simulink model "servopositioner"  (R2015b)
settings: Solver=ode45  StartTime=0.0  StopTime=100  RelTol=1e-3
values from neighbouring files (symbols this model uses):
  Aa = pi*(Dp^2)/4    (= 0.00020106192983)    [param_JOB.m]
  Ab = pi*(Dp^2-Dr^2)/4    (= 0.00012252211349)    [param_JOB.m]
  acc = 0    [param_JOB.m]
  beta = 1.4e9    (= 1400000000)    [param_JOB.m]
  fv = 700    [param_JOB.m]
  In = 10e-3    (= 0.01)    [param_JOB.m]
  Kva = Kv*sqrt(2)    [param_JOB.m]
  Kvb = Kv*sqrt(2)    [param_JOB.m]
  KvlkA = Kvlk    [param_JOB.m]
  KvlkB = Kvlk    [param_JOB.m]
  L = 0.5    [beta_hose_calc.m]    (also in param_JOB.m = 0.08)
  leak = 0    [param_JOB.m]
  lw_dz = 0    [param_JOB.m]
  Mp = ((pi*Dr^2/4)*L + Aa*0.15)*7860    (= 0.286437851784)    [param_JOB.m]
  n = 1.4    [beta_hose_calc.m]    (also in beta_w_air_entrance.m; param_JOB.m)
  P0 = 100e5    (= 10000000)    [beta_hose_calc.m]    (also in param_JOB.m)
  pAo = ps/2    (= 8000000)    [param_JOB.m]
  pBo = ps/2    (= 8000000)    [param_JOB.m]
  ps = 1e5:1e5:120e5    [beta_w_air_entrance.m]    (also in param_JOB.m = 16000000)
  pt = 10e5    (= 1000000)    [param_JOB.m]
  up_dz = 0    [param_JOB.m]
  V0 = A*L    (= 6.13592315154e-05)    [beta_hose_calc.m]    (also in param_JOB.m = 4e-05)
  V0A = v1a + v2a    (= 2.90341084306e-06)    [param_JOB.m]
  V0B = v1b + v2b + v3b    (= 1.67615552692e-06)    [param_JOB.m]
  wn = 2*100*pi    (= 628.318530718)    [param_JOB.m]
libraries: simulink x2
settings Model: Creator=Toshiba  LastModifiedBy=Toshiba
settings SolverCC: ZeroCrossAlgorithm=Adaptive
settings DataIOCC: SaveFormat=Array
settings DebuggingCC: UnderspecifiedInitializationDetection=Classic  MergeDetectMultiDrivingBlocksExec=none  SolverPrmCheckMsg=warning  StateNameClashWarn=warning
settings HardwareCC: ProdBitPerPointer=32  ProdLargestAtomicFloat=None  ProdIntDivRoundTo=Undefined  ProdEndianess=Unspecified  ProdWordSize=32  ProdHWDeviceType=32-bit Generic
settings GRTTargetCC: GeneratePreprocessorConditionals=Disable all
settings ConfigComp: CovModelRefEnable=Off

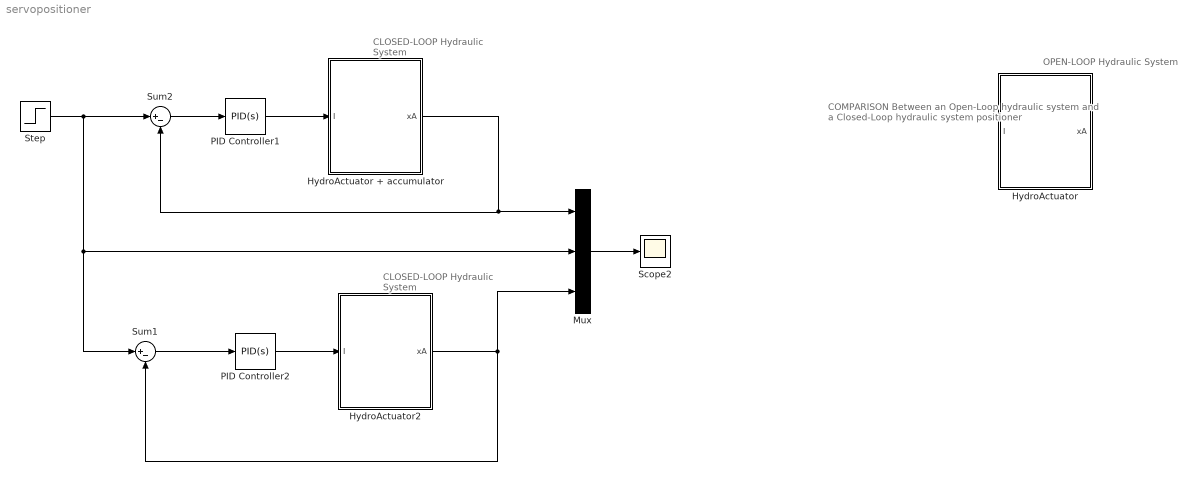
== system servopositioner ==
  note: OPEN-LOOP
      | Hydraulic System
  note: COMPARISON Between
      | an Open-Loop hydraulic system
      | and a Closed-Loop hydraulic
      | system positioner
  note: CLOSED-LOOP
      | Hydraulic System
  note: CLOSED-LOOP
      | Hydraulic System
  HydroActuator : Subsystem
  HydroActuator + accumulator : Subsystem
  HydroActuator2 : Subsystem
  Mux : Mux  Inputs=3
  PID Controller1 : simulink/Continuous/PID Controller  Controller=PID  TimeDomain=Continuous-time  SampleTime=-1  IntegratorMethod=Forward Euler  FilterMethod=Forward Euler  Form=Parallel  UseFilter=on  ControllerParametersSource=internal  P=700  I=50  D=0  N=100  InitialConditionSource=internal  InitialConditionForIntegrator=0  InitialConditionForFilter=0  ExternalReset=none  LimitOutput=off  UpperSaturationLimit=inf  LowerSaturationLimit=-inf  LinearizeAsGain=on  AntiWindupMode=none  Kb=1  TrackingMode=off  Kt=1  PParamMin=[]  PParamMax=[]  IParamMin=[]  IParamMax=[]  DParamMin=[]  DParamMax=[]  NParamMin=[]  NParamMax=[]  KbParamMin=[]  KbParamMax=[]  KtParamMin=[]  KtParamMax=[]  POutMin=[]  POutMax=[]  IOutMin=[]  IOutMax=[]  DOutMin=[]  DOutMax=[]  NOutMin=[]  NOutMax=[]  KbOutMin=[]  KbOutMax=[]  KtOutMin=[]  KtOutMax=[]  IntegratorOutMin=[]  IntegratorOutMax=[]  FilterOutMin=[]  FilterOutMax=[]  SumOutMin=[]  SumOutMax=[]  SumI1OutMin=[]  SumI1OutMax=[]  SumI2OutMin=[]  SumI2OutMax=[]  SumI3OutMin=[]  SumI3OutMax=[]  SumDOutMin=[]  SumDOutMax=[]  SaturationOutMin=[]  SaturationOutMax=[]  IntegratorContinuousStateAttributes=''  IntegratorStateMustResolveToSignalObject=off  IntegratorRTWStateStorageClass=Auto  FilterContinuousStateAttributes=''  FilterStateMustResolveToSignalObject=off  FilterRTWStateStorageClass=Auto  DifferentiatorICPrevScaledInput=0  DifferentiatorOutMin=[]  DifferentiatorOutMax=[]
  PID Controller2 : simulink/Continuous/PID Controller  Controller=PID  TimeDomain=Continuous-time  SampleTime=-1  IntegratorMethod=Forward Euler  FilterMethod=Forward Euler  Form=Parallel  UseFilter=on  ControllerParametersSource=internal  P=700  I=50  D=0  N=100  InitialConditionSource=internal  InitialConditionForIntegrator=0  InitialConditionForFilter=0  ExternalReset=none  LimitOutput=off  UpperSaturationLimit=inf  LowerSaturationLimit=-inf  LinearizeAsGain=on  AntiWindupMode=none  Kb=1  TrackingMode=off  Kt=1  PParamMin=[]  PParamMax=[]  IParamMin=[]  IParamMax=[]  DParamMin=[]  DParamMax=[]  NParamMin=[]  NParamMax=[]  KbParamMin=[]  KbParamMax=[]  KtParamMin=[]  KtParamMax=[]  POutMin=[]  POutMax=[]  IOutMin=[]  IOutMax=[]  DOutMin=[]  DOutMax=[]  NOutMin=[]  NOutMax=[]  KbOutMin=[]  KbOutMax=[]  KtOutMin=[]  KtOutMax=[]  IntegratorOutMin=[]  IntegratorOutMax=[]  FilterOutMin=[]  FilterOutMax=[]  SumOutMin=[]  SumOutMax=[]  SumI1OutMin=[]  SumI1OutMax=[]  SumI2OutMin=[]  SumI2OutMax=[]  SumI3OutMin=[]  SumI3OutMax=[]  SumDOutMin=[]  SumDOutMax=[]  SaturationOutMin=[]  SaturationOutMax=[]  IntegratorContinuousStateAttributes=''  IntegratorStateMustResolveToSignalObject=off  IntegratorRTWStateStorageClass=Auto  FilterContinuousStateAttributes=''  FilterStateMustResolveToSignalObject=off  FilterRTWStateStorageClass=Auto  DifferentiatorICPrevScaledInput=0  DifferentiatorOutMin=[]  DifferentiatorOutMax=[]
  Scope2 : Scope
  Step : Step  Time=3  After=0.04  SampleTime=0
  Sum1 : Sum  Inputs=|+-
  Sum2 : Sum  Inputs=|+-
  wires:
  Step/1 -> Sum2/1, Mux/2, Sum1/1
  PID Controller1/1 -> HydroActuator + accumulator/1(I)
  Mux/1 -> Scope2/1
  HydroActuator2/1(xA) -> Mux/3, Sum1/2
  Sum1/1 -> PID Controller2/1
  PID Controller2/1 -> HydroActuator2/1(I)
  Sum2/1 -> PID Controller1/1
  HydroActuator + accumulator/1(xA) -> Sum2/2, Mux/1

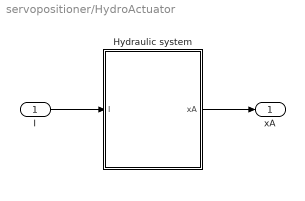
== system servopositioner/HydroActuator ==
  I : Inport
  Hydraulic system : Subsystem
  xA : Outport
  wires:
  I/1 -> Hydraulic system/1(I)
  Hydraulic system/1(xA) -> xA/1

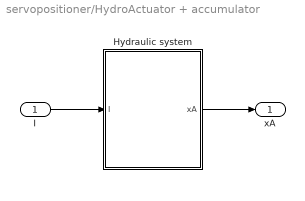
== system servopositioner/HydroActuator + accumulator ==
  I : Inport
  Hydraulic system : Subsystem
  xA : Outport
  wires:
  Hydraulic system/1(xA) -> xA/1
  I/1 -> Hydraulic system/1(I)

== system servopositioner/HydroActuator2 ==
  I : Inport
  Hydraulic system : Subsystem
  xA : Outport
  wires:
  I/1 -> Hydraulic system/1(I)
  Hydraulic system/1(xA) -> xA/1

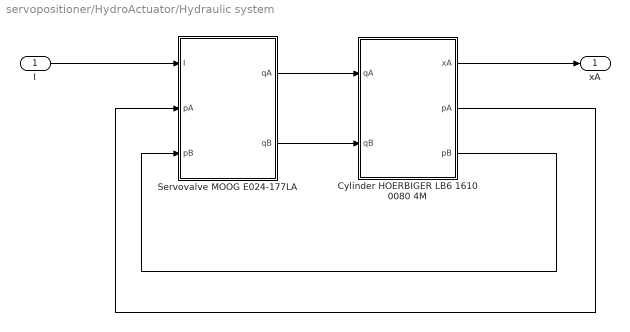
== system servopositioner/HydroActuator/Hydraulic system ==
  I : Inport
  Cylinder HOERBIGER LB6 1610 0080 4M : Subsystem
  Servovalve MOOG E024-177LA : Subsystem
  xA : Outport
  wires:
  Servovalve MOOG E024-177LA/2(qB) -> Cylinder HOERBIGER LB6 1610 0080 4M/2(qB)
  Servovalve MOOG E024-177LA/1(qA) -> Cylinder HOERBIGER LB6 1610 0080 4M/1(qA)
  Cylinder HOERBIGER LB6 1610 0080 4M/2(pA) -> Servovalve MOOG E024-177LA/2(pA)
  Cylinder HOERBIGER LB6 1610 0080 4M/3(pB) -> Servovalve MOOG E024-177LA/3(pB)
  I/1 -> Servovalve MOOG E024-177LA/1(I)
  Cylinder HOERBIGER LB6 1610 0080 4M/1(xA) -> xA/1

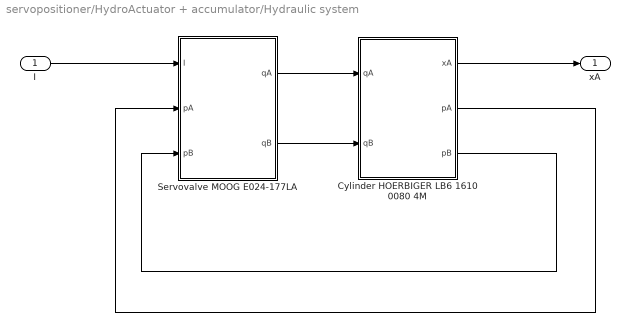
== system servopositioner/HydroActuator + accumulator/Hydraulic system ==
  I : Inport
  Cylinder HOERBIGER LB6 1610 0080 4M : Subsystem
  Servovalve MOOG E024-177LA : Subsystem
  xA : Outport
  wires:
  Cylinder HOERBIGER LB6 1610 0080 4M/1(xA) -> xA/1
  I/1 -> Servovalve MOOG E024-177LA/1(I)
  Cylinder HOERBIGER LB6 1610 0080 4M/3(pB) -> Servovalve MOOG E024-177LA/3(pB)
  Cylinder HOERBIGER LB6 1610 0080 4M/2(pA) -> Servovalve MOOG E024-177LA/2(pA)
  Servovalve MOOG E024-177LA/1(qA) -> Cylinder HOERBIGER LB6 1610 0080 4M/1(qA)
  Servovalve MOOG E024-177LA/2(qB) -> Cylinder HOERBIGER LB6 1610 0080 4M/2(qB)

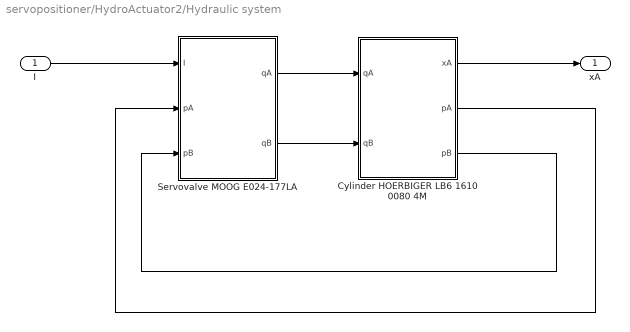
== system servopositioner/HydroActuator2/Hydraulic system ==
  I : Inport
  Cylinder HOERBIGER LB6 1610 0080 4M : Subsystem
  Servovalve MOOG E024-177LA : Subsystem
  xA : Outport
  wires:
  Servovalve MOOG E024-177LA/2(qB) -> Cylinder HOERBIGER LB6 1610 0080 4M/2(qB)
  Servovalve MOOG E024-177LA/1(qA) -> Cylinder HOERBIGER LB6 1610 0080 4M/1(qA)
  Cylinder HOERBIGER LB6 1610 0080 4M/2(pA) -> Servovalve MOOG E024-177LA/2(pA)
  Cylinder HOERBIGER LB6 1610 0080 4M/3(pB) -> Servovalve MOOG E024-177LA/3(pB)
  I/1 -> Servovalve MOOG E024-177LA/1(I)
  Cylinder HOERBIGER LB6 1610 0080 4M/1(xA) -> xA/1

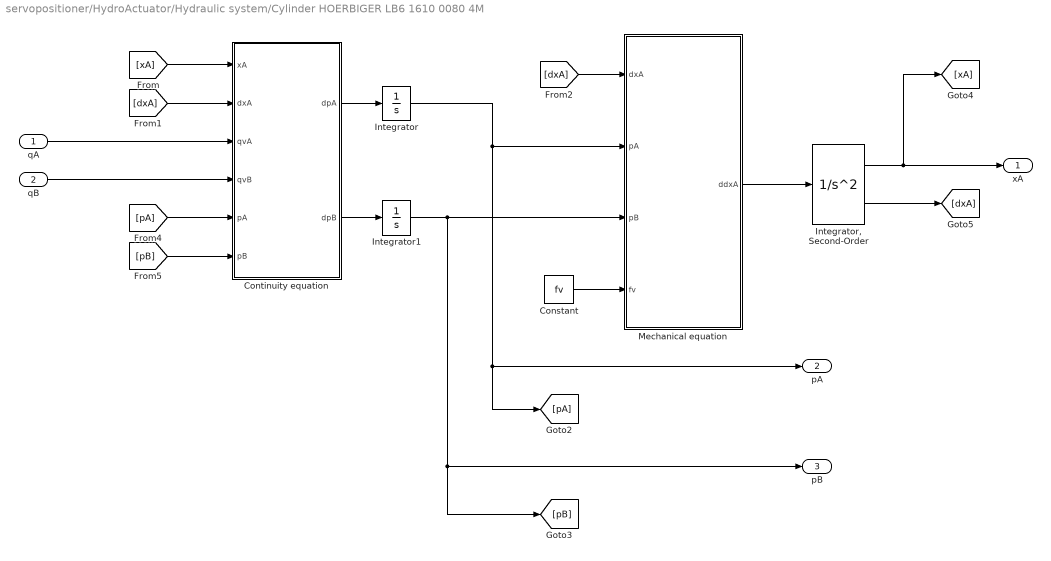
== system servopositioner/HydroActuator/Hydraulic system/Cylinder HOERBIGER LB6 1610 0080 4M ==
  qA : Inport
  qB : Inport  Port=2
  Constant : Constant  Value=fv
  Continuity equation : MATLAB Function  TreatAsAtomicUnit=on
  Integrator : Integrator  InitialCondition=pAo
  "Integrator, Second-Order" : SecondOrderIntegrator  ICX=xo  LimitX=on  UpperLimitX=L  LowerLimitX=0
  Integrator1 : Integrator  InitialCondition=pBo
  Mechanical equation : MATLAB Function  TreatAsAtomicUnit=on
  xA : Outport
  pA : Outport  Port=2
  pB : Outport  Port=3
  wires:
  Continuity equation/1(dpA) -> Integrator/1
  Continuity equation/2(dpB) -> Integrator1/1
  qA/1 -> Continuity equation/3(qvA)
  qB/1 -> Continuity equation/4(qvB)
  [dxA] -> Continuity equation/2(dxA)
  [xA] -> Continuity equation/1(xA)
  Constant/1 -> Mechanical equation/4(fv)
  [dxA] -> Mechanical equation/1(dxA)
  Integrator/1 -> [pA], pA/1, Mechanical equation/2(pA)
  Integrator1/1 -> [pB], pB/1, Mechanical equation/3(pB)
  [pA] -> Continuity equation/5(pA)
  [pB] -> Continuity equation/6(pB)
  Mechanical equation/1(ddxA) -> "Integrator, Second-Order"/1
  "Integrator, Second-Order"/1 -> xA/1, [xA]
  "Integrator, Second-Order"/2 -> [dxA]

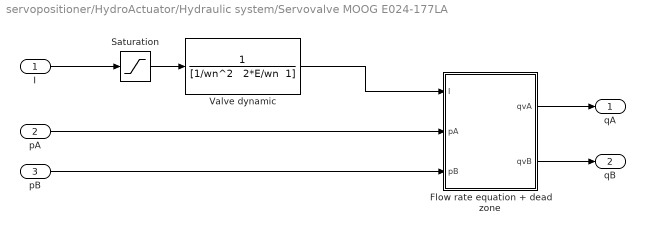
== system servopositioner/HydroActuator/Hydraulic system/Servovalve MOOG E024-177LA ==
  I : Inport
  pA : Inport  Port=2
  pB : Inport  Port=3
  Flow rate equation + dead zone : MATLAB Function  TreatAsAtomicUnit=on
  Saturation : Saturate  UpperLimit=In  LowerLimit=-In  LinearizeAsGain=off
  Valve dynamic : TransferFcn  Numerator=1  Denominator="[1/wn^2   2*E/wn  1]"
  qA : Outport
  qB : Outport  Port=2
  wires:
  Saturation/1 -> Valve dynamic/1
  I/1 -> Saturation/1
  Valve dynamic/1 -> Flow rate equation + dead zone/1(I)
  pA/1 -> Flow rate equation + dead zone/2(pA)
  pB/1 -> Flow rate equation + dead zone/3(pB)
  Flow rate equation + dead zone/2(qvB) -> qB/1
  Flow rate equation + dead zone/1(qvA) -> qA/1

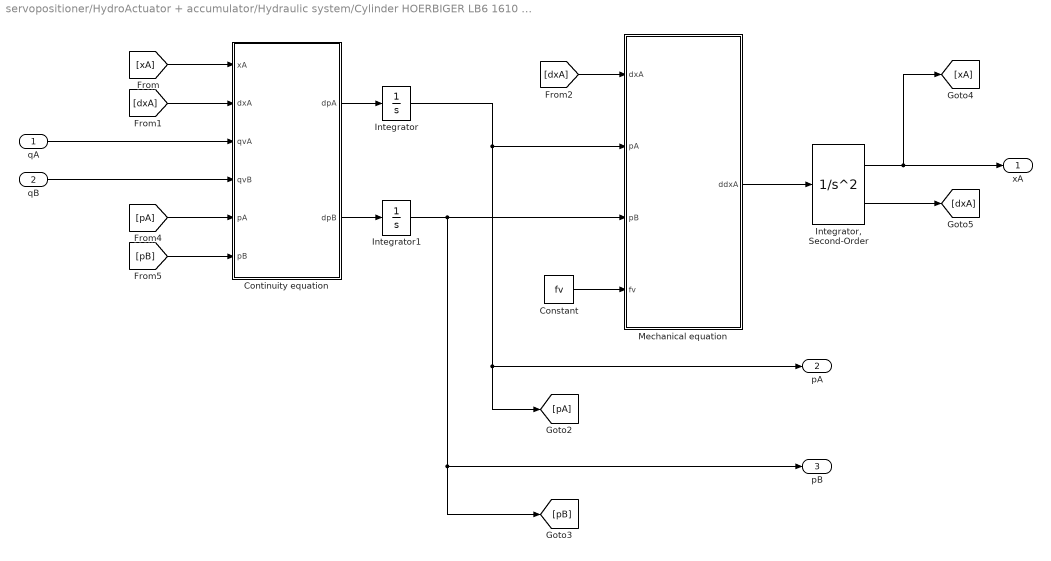
== system servopositioner/HydroActuator + accumulator/Hydraulic system/Cylinder HOERBIGER LB6 1610 0080 4M ==
  qA : Inport
  qB : Inport  Port=2
  Constant : Constant  Value=fv
  Continuity equation : MATLAB Function  TreatAsAtomicUnit=on
  Integrator : Integrator  InitialCondition=pAo
  "Integrator, Second-Order" : SecondOrderIntegrator  ICX=xo  LimitX=on  UpperLimitX=L  LowerLimitX=0
  Integrator1 : Integrator  InitialCondition=pBo
  Mechanical equation : MATLAB Function  TreatAsAtomicUnit=on
  xA : Outport
  pA : Outport  Port=2
  pB : Outport  Port=3
  wires:
  "Integrator, Second-Order"/2 -> [dxA]
  "Integrator, Second-Order"/1 -> [xA], xA/1
  Mechanical equation/1(ddxA) -> "Integrator, Second-Order"/1
  [pB] -> Continuity equation/6(pB)
  [pA] -> Continuity equation/5(pA)
  Integrator1/1 -> Mechanical equation/3(pB), pB/1, [pB]
  Integrator/1 -> Mechanical equation/2(pA), pA/1, [pA]
  [dxA] -> Mechanical equation/1(dxA)
  Constant/1 -> Mechanical equation/4(fv)
  [xA] -> Continuity equation/1(xA)
  [dxA] -> Continuity equation/2(dxA)
  qB/1 -> Continuity equation/4(qvB)
  qA/1 -> Continuity equation/3(qvA)
  Continuity equation/2(dpB) -> Integrator1/1
  Continuity equation/1(dpA) -> Integrator/1

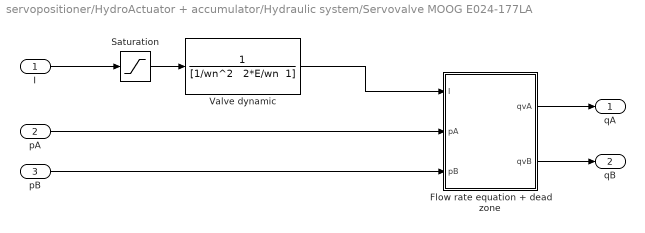
== system servopositioner/HydroActuator + accumulator/Hydraulic system/Servovalve MOOG E024-177LA ==
  I : Inport
  pA : Inport  Port=2
  pB : Inport  Port=3
  Flow rate equation + dead zone : MATLAB Function  TreatAsAtomicUnit=on
  Saturation : Saturate  UpperLimit=In  LowerLimit=-In  LinearizeAsGain=off
  Valve dynamic : TransferFcn  Numerator=1  Denominator="[1/wn^2   2*E/wn  1]"
  qA : Outport
  qB : Outport  Port=2
  wires:
  Flow rate equation + dead zone/1(qvA) -> qA/1
  Flow rate equation + dead zone/2(qvB) -> qB/1
  pB/1 -> Flow rate equation + dead zone/3(pB)
  pA/1 -> Flow rate equation + dead zone/2(pA)
  Valve dynamic/1 -> Flow rate equation + dead zone/1(I)
  I/1 -> Saturation/1
  Saturation/1 -> Valve dynamic/1

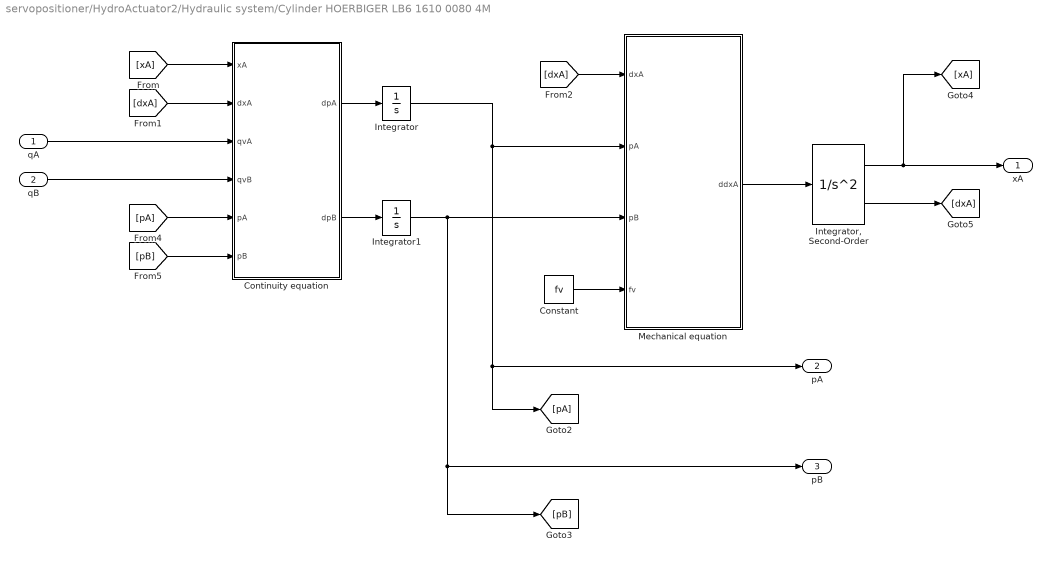
== system servopositioner/HydroActuator2/Hydraulic system/Cylinder HOERBIGER LB6 1610 0080 4M ==
  qA : Inport
  qB : Inport  Port=2
  Constant : Constant  Value=fv
  Continuity equation : MATLAB Function  TreatAsAtomicUnit=on
  Integrator : Integrator  InitialCondition=pAo
  "Integrator, Second-Order" : SecondOrderIntegrator  ICX=xo  LimitX=on  UpperLimitX=L  LowerLimitX=0
  Integrator1 : Integrator  InitialCondition=pBo
  Mechanical equation : MATLAB Function  TreatAsAtomicUnit=on
  xA : Outport
  pA : Outport  Port=2
  pB : Outport  Port=3
  wires:
  Continuity equation/1(dpA) -> Integrator/1
  Continuity equation/2(dpB) -> Integrator1/1
  qA/1 -> Continuity equation/3(qvA)
  qB/1 -> Continuity equation/4(qvB)
  [dxA] -> Continuity equation/2(dxA)
  [xA] -> Continuity equation/1(xA)
  Constant/1 -> Mechanical equation/4(fv)
  [dxA] -> Mechanical equation/1(dxA)
  Integrator/1 -> [pA], pA/1, Mechanical equation/2(pA)
  Integrator1/1 -> [pB], pB/1, Mechanical equation/3(pB)
  [pA] -> Continuity equation/5(pA)
  [pB] -> Continuity equation/6(pB)
  Mechanical equation/1(ddxA) -> "Integrator, Second-Order"/1
  "Integrator, Second-Order"/1 -> xA/1, [xA]
  "Integrator, Second-Order"/2 -> [dxA]

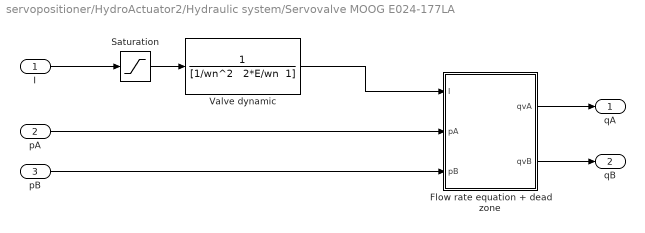
== system servopositioner/HydroActuator2/Hydraulic system/Servovalve MOOG E024-177LA ==
  I : Inport
  pA : Inport  Port=2
  pB : Inport  Port=3
  Flow rate equation + dead zone : MATLAB Function  TreatAsAtomicUnit=on
  Saturation : Saturate  UpperLimit=In  LowerLimit=-In  LinearizeAsGain=off
  Valve dynamic : TransferFcn  Numerator=1  Denominator="[1/wn^2   2*E/wn  1]"
  qA : Outport
  qB : Outport  Port=2
  wires:
  Saturation/1 -> Valve dynamic/1
  I/1 -> Saturation/1
  Valve dynamic/1 -> Flow rate equation + dead zone/1(I)
  pA/1 -> Flow rate equation + dead zone/2(pA)
  pB/1 -> Flow rate equation + dead zone/3(pB)
  Flow rate equation + dead zone/2(qvB) -> qB/1
  Flow rate equation + dead zone/1(qvA) -> qA/1

== matlab function servopositioner/HydroActuator + accumulator/Hydraulic system/Cylinder HOERBIGER LB6 1610 0080 4M/Continuity equation ==
  data: xA input; dpA output; dpB output; dxA input; qvA input; qvB input; pA input; pB input; leak parameter; V0A parameter; V0B parameter; Aa parameter; Ab parameter; L parameter; beta parameter; n parameter; V0 parameter; P0 parameter
function [dpA,dpB] = fcn(xA, dxA, qvA, qvB, pA, pB, leak, V0A, V0B, Aa, Ab, L, beta, n, V0, P0)

pC = pA - pB;   % Pressao de carga [Pa]

qvlk = leak * pC;
  
CA_A  = (V0A + Aa*xA) / beta;                      % Capacitancia hidráulica do atuador [m^3/Pa]
CAC_A = (V0*P0^(1/n))/(n* (pA+1e5)^((n+1)/n));     % Capacitancia hidráulica do acumulador [m^3/Pa]
CA_B  = (V0B + Ab*(L-xA)) / beta;                  % Capacitancia hidráulica do atuador [m^3/Pa]
CAC_B = (V0*P0^(1/n))/(n* (pB+1e5)^((n+1)/n));     % Capacitancia hidráulica do acumulador [m^3/Pa]

CT_A  = CA_A + CAC_A;                              % Capacitancia total em A
CT_B  = CA_B + CAC_B;                              % Capacitancia total em B 

%       /        \
%       |   1    | /                    \
% dpA = | ------ | | qvA - Aa*dx - qvex | 
%       |  CT_A  | \                    /
%       \        /
      
dpA = CT_A^-1 * (qvA - Aa*dxA - qvlk);

%       /        \
%       |   1    | /                    \
% dpB = | ------ | | Ab*dx + qvex - qvB | 
%       |  CT_B  | \                    /
%       \        /
      
dpB = CT_B^-1 * (Ab*dxA + qvlk - qvB);

== matlab function servopositioner/HydroActuator + accumulator/Hydraulic system/Cylinder HOERBIGER LB6 1610 0080 4M/Mechanical equation ==
  data: ddxA output; dxA input; pA input; pB input; fv input; Aa parameter; Ab parameter; Mp parameter
function ddxA = fcn(dxA, pA, pB, fv, Aa, Ab, Mp)
%#codegen

FH  = pA*Aa - pB*Ab;     % N - Hydraulic force
Ffr = fv*dxA;            % N - Friction force (Viscous)
ddxA  = (FH - Ffr)/Mp;     % m/s2 - Acceleration

== matlab function servopositioner/HydroActuator/Hydraulic system/Cylinder HOERBIGER LB6 1610 0080 4M/Continuity equation ==
  data: xA input; dpA output; dpB output; dxA input; qvA input; qvB input; pA input; pB input; leak parameter; V0A parameter; V0B parameter; Aa parameter; Ab parameter; L parameter; beta parameter; n parameter; V0 parameter; P0 parameter; acc parameter
function [dpA,dpB] = fcn(xA, dxA, qvA, qvB, pA, pB, leak, V0A, V0B, Aa, Ab, L, beta, n, V0, P0, acc)

pC = pA - pB;   % Pressao de carga [Pa]

qvlk = leak * pC;
dpa = 0;
dpb = 0;

if acc == 0,
%       /              \
%       |     beta     | /                    \
% dpA = | ------------ | | qvA - Aa*dx - qvex | 
%       |  Va0 + Aa*x  | \                    /
%       \              /
      
dpa = (beta/(V0A + Aa*xA)) * (qvA - Aa*dxA - qvlk);

%       /                  \
%       |     beta         | /                    \
% dpB = | ---------------- | | Ab*dx + qvex - qvB | 
%       | Vb0 + Ab*(L - x) | \                    /
%       \                  /
      
dpb = (beta/(V0B + Ab*(L-xA))) * (Ab*dxA + qvlk - qvB);

elseif acc == 1,
    
CA_A  = (V0A + Aa*xA) / beta;                      % Capacitancia hidráulica do atuador [m^3/Pa]
CAC_A = (V0*P0^(1/n))/(n* (pA+1e5)^((n+1)/n));     % Capacitancia hidráulica do acumulador [m^3/Pa]
CA_B  = (V0B + Ab*(L-xA)) / beta;                  % Capacitancia hidráulica do atuador [m^3/Pa]
CAC_B = (V0*P0^(1/n))/(n* (pB+1e5)^((n+1)/n));     % Capacitancia hidráulica do acumulador [m^3/Pa]

CT_A  = CA_A + CAC_A;                              % Capacitancia total em A
CT_B  = CA_B + CAC_B;                              % Capacitancia total em B 


%       /        \
%       |   1    | /                    \
% dpA = | ------ | | qvA - Aa*dx - qvex | 
%       |  CT_A  | \                    /
%       \        /
      
dpa = CT_A^-1 * (qvA - Aa*dxA - qvlk);

%       /        \
%       |   1    | /                    \
% dpB = | ------ | | Ab*dx + qvex - qvB | 
%       |  CT_B  | \                    /
%       \        /
      
dpb = CT_B^-1 * (Ab*dxA + qvlk - qvB);
end

dpA = dpa;
dpB = dpb;

== matlab function servopositioner/HydroActuator/Hydraulic system/Cylinder HOERBIGER LB6 1610 0080 4M/Mechanical equation ==
  data: ddxA output; dxA input; pA input; pB input; fv input; Aa parameter; Ab parameter; Mp parameter
function ddxA = fcn(dxA, pA, pB, fv, Aa, Ab, Mp)
%#codegen

FH  = pA*Aa - pB*Ab;     % N - Hydraulic force
Ffr = fv*dxA;            % N - Friction force (Viscous)
ddxA  = (FH - Ffr)/Mp;     % m/s2 - Acceleration

== matlab function servopositioner/HydroActuator + accumulator/Hydraulic system/Servovalve MOOG E024-177LA/Flow rate equation + dead zone ==
  data I settings: updateMethod=SF_CONTINUOUS_TIME_DATA
  data qvA settings: updateMethod=SF_CONTINUOUS_TIME_DATA
  data qvB settings: updateMethod=SF_CONTINUOUS_TIME_DATA
  data: I input; qvA output; qvB output; In parameter; Kva parameter; Kvb parameter; KvlkA parameter; KvlkB parameter; up_dz parameter; lw_dz parameter; ps parameter; pt parameter; pA input; pB input
function [qvA , qvB] = fcn(I, In, Kva, Kvb, KvlkA, KvlkB,up_dz, lw_dz, ps, pt, pA, pB)

if (I>=up_dz) && (I<=In),
    qvA = (Kva*(I/In) + KvlkA) * sign(ps-pA)*sqrt(abs(ps-pA)) - KvlkA*sign(pA-pt)*sqrt(abs(pA-pt)) ;
    qvB = (Kvb*(I/In) + KvlkB) * sign(pB-pt)*sqrt(abs(pB-pt)) - KvlkB*sign(ps-pB)*sqrt(abs(ps-pB)) ;
elseif (I>=-In) && (I<=lw_dz), 
    qvA = KvlkA*sign(ps-pA)*sqrt(abs(ps-pA)) - (Kva*(abs(I)/In) + KvlkA) * sign(pA-pt)*sqrt(abs(pA-pt));
     qvB = KvlkB*sign(pB-pt)*sqrt(abs(pB-pt)) - (Kvb*(abs(I)/In) + KvlkB) * sign(ps-pB)*sqrt(abs(ps-pB));
else
    qvA = 0;
    qvB = 0;
end
end

== matlab function servopositioner/HydroActuator/Hydraulic system/Servovalve MOOG E024-177LA/Flow rate equation + dead zone ==
  data I settings: updateMethod=SF_CONTINUOUS_TIME_DATA
  data qvA settings: updateMethod=SF_CONTINUOUS_TIME_DATA
  data qvB settings: updateMethod=SF_CONTINUOUS_TIME_DATA
  data: I input; qvA output; qvB output; In parameter; Kva parameter; Kvb parameter; KvlkA parameter; KvlkB parameter; up_dz parameter; lw_dz parameter; ps parameter; pt parameter; pA input; pB input
function [qvA , qvB] = fcn(I, In, Kva, Kvb, KvlkA, KvlkB,up_dz, lw_dz, ps, pt, pA, pB)

if (I>=up_dz) && (I<=In),
    qvA = (Kva*(I/In) + KvlkA) * sign(ps-pA)*sqrt(abs(ps-pA)) - KvlkA*sign(pA-pt)*sqrt(abs(pA-pt)) ;
    qvB = (Kvb*(I/In) + KvlkB) * sign(pB-pt)*sqrt(abs(pB-pt)) - KvlkB*sign(ps-pB)*sqrt(abs(ps-pB)) ;
elseif (I>=-In) && (I<=lw_dz), 
    qvA = KvlkA*sign(ps-pA)*sqrt(abs(ps-pA)) - (Kva*(abs(I)/In) + KvlkA) * sign(pA-pt)*sqrt(abs(pA-pt));
     qvB = KvlkB*sign(pB-pt)*sqrt(abs(pB-pt)) - (Kvb*(abs(I)/In) + KvlkB) * sign(ps-pB)*sqrt(abs(ps-pB));
else
    qvA = 0;
    qvB = 0;
end
end

== matlab function servopositioner/HydroActuator2/Hydraulic system/Cylinder HOERBIGER LB6 1610 0080 4M/Continuity equation ==
  data: xA input; dpA output; dpB output; dxA input; qvA input; qvB input; pA input; pB input; leak parameter; V0A parameter; V0B parameter; Aa parameter; Ab parameter; L parameter; beta parameter; n parameter; V0 parameter; P0 parameter; acc parameter
function [dpA,dpB] = fcn(xA, dxA, qvA, qvB, pA, pB, leak, V0A, V0B, Aa, Ab, L, beta, n, V0, P0, acc)

pC = pA - pB;   % Pressao de carga [Pa]

qvlk = leak * pC;
dpa = 0;
dpb = 0;

if acc == 0,
%       /              \
%       |     beta     | /                    \
% dpA = | ------------ | | qvA - Aa*dx - qvex | 
%       |  Va0 + Aa*x  | \                    /
%       \              /
      
dpa = (beta/(V0A + Aa*xA)) * (qvA - Aa*dxA - qvlk);

%       /                  \
%       |     beta         | /                    \
% dpB = | ---------------- | | Ab*dx + qvex - qvB | 
%       | Vb0 + Ab*(L - x) | \                    /
%       \                  /
      
dpb = (beta/(V0B + Ab*(L-xA))) * (Ab*dxA + qvlk - qvB);

elseif acc == 1,
    
CA_A  = (V0A + Aa*xA) / beta;                      % Capacitancia hidráulica do atuador [m^3/Pa]
CAC_A = (V0*P0^(1/n))/(n* (pA+1e5)^((n+1)/n));     % Capacitancia hidráulica do acumulador [m^3/Pa]
CA_B  = (V0B + Ab*(L-xA)) / beta;                  % Capacitancia hidráulica do atuador [m^3/Pa]
CAC_B = (V0*P0^(1/n))/(n* (pB+1e5)^((n+1)/n));     % Capacitancia hidráulica do acumulador [m^3/Pa]

CT_A  = CA_A + CAC_A;                              % Capacitancia total em A
CT_B  = CA_B + CAC_B;                              % Capacitancia total em B 


%       /        \
%       |   1    | /                    \
% dpA = | ------ | | qvA - Aa*dx - qvex | 
%       |  CT_A  | \                    /
%       \        /
      
dpa = CT_A^-1 * (qvA - Aa*dxA - qvlk);

%       /        \
%       |   1    | /                    \
% dpB = | ------ | | Ab*dx + qvex - qvB | 
%       |  CT_B  | \                    /
%       \        /
      
dpb = CT_B^-1 * (Ab*dxA + qvlk - qvB);
end

dpA = dpa;
dpB = dpb;

== matlab function servopositioner/HydroActuator2/Hydraulic system/Cylinder HOERBIGER LB6 1610 0080 4M/Mechanical equation ==
  data: ddxA output; dxA input; pA input; pB input; fv input; Aa parameter; Ab parameter; Mp parameter
function ddxA = fcn(dxA, pA, pB, fv, Aa, Ab, Mp)
%#codegen

FH  = pA*Aa - pB*Ab;     % N - Hydraulic force
Ffr = fv*dxA;            % N - Friction force (Viscous)
ddxA  = (FH - Ffr)/Mp;     % m/s2 - Acceleration

== matlab function servopositioner/HydroActuator2/Hydraulic system/Servovalve MOOG E024-177LA/Flow rate equation + dead zone ==
  data I settings: updateMethod=SF_CONTINUOUS_TIME_DATA
  data qvA settings: updateMethod=SF_CONTINUOUS_TIME_DATA
  data qvB settings: updateMethod=SF_CONTINUOUS_TIME_DATA
  data: I input; qvA output; qvB output; In parameter; Kva parameter; Kvb parameter; KvlkA parameter; KvlkB parameter; up_dz parameter; lw_dz parameter; ps parameter; pt parameter; pA input; pB input
function [qvA , qvB] = fcn(I, In, Kva, Kvb, KvlkA, KvlkB,up_dz, lw_dz, ps, pt, pA, pB)

if (I>=up_dz) && (I<=In),
    qvA = (Kva*(I/In) + KvlkA) * sign(ps-pA)*sqrt(abs(ps-pA)) - KvlkA*sign(pA-pt)*sqrt(abs(pA-pt)) ;
    qvB = (Kvb*(I/In) + KvlkB) * sign(pB-pt)*sqrt(abs(pB-pt)) - KvlkB*sign(ps-pB)*sqrt(abs(ps-pB)) ;
elseif (I>=-In) && (I<=lw_dz), 
    qvA = KvlkA*sign(ps-pA)*sqrt(abs(ps-pA)) - (Kva*(abs(I)/In) + KvlkA) * sign(pA-pt)*sqrt(abs(pA-pt));
     qvB = KvlkB*sign(pB-pt)*sqrt(abs(pB-pt)) - (Kvb*(abs(I)/In) + KvlkB) * sign(ps-pB)*sqrt(abs(ps-pB));
else
    qvA = 0;
    qvB = 0;
end
end
